simulink model "project"  (R2022b)
settings: Solver=ode15s  StartTime=0.0  StopTime=2  RelTol=1e-3
libraries: spsSeriesRLCBranchLib x6, spsVoltageMeasurementLib x4, spsCurrentMeasurementLib x3, spsFullBridgeMMCExternalDCLinksLib x1, spsOnDelayLib x1, spsPVArrayLib x1, spsPWMGeneratorMultilevelLib x1, spsDiodeLib x1, spsMosfetLib x1, spspowerguiLib x1
settings Model: Creator=nisha  LastModifiedBy=nisha

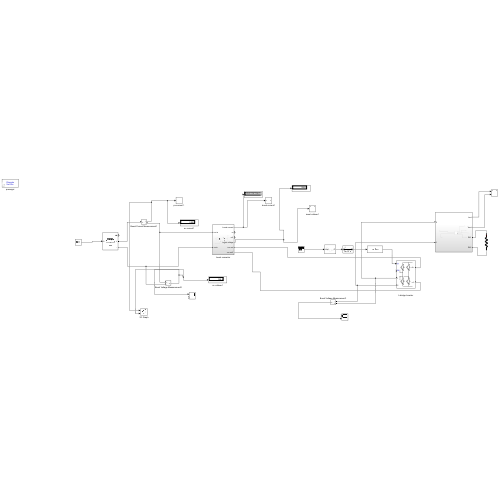
[thumbnail: Simulink's stored preview of the top-level diagram]
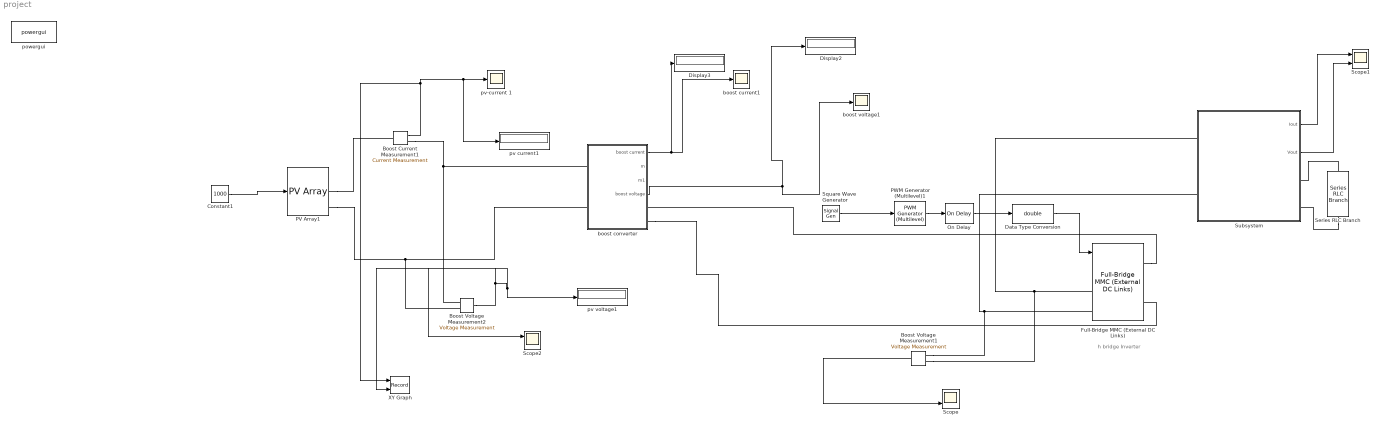
== system project ==
  note: h bridge Inverter
  Boost Current Measurement1 : spsCurrentMeasurementLib/Current Measurement  PhasorSimulation=off  OutputType=Complex  PSBequivalent=0
  Boost Voltage Measurement1 : spsVoltageMeasurementLib/Voltage Measurement  PhasorSimulation=off  OutputType=Complex  PSBequivalent=0
  Boost Voltage Measurement2 : spsVoltageMeasurementLib/Voltage Measurement  PhasorSimulation=off  OutputType=Complex  PSBequivalent=0
  Constant1 : Constant  Value=1000
  Data Type Conversion : DataTypeConversion  OutDataTypeStr=double  SaturateOnIntegerOverflow=off  RndMeth=Floor
  Display2 : Display
  Display3 : Display
      settings: Format=long_e
  Full-Bridge MMC (External DC Links) : spsFullBridgeMMCExternalDCLinksLib/Full-Bridge MMC (External DC Links)  ModelType=Switching devices  n=1  Ron=1e-3  Rs=1e6  Cs=inf  Ron_Diode=1e-3  Rs_Diode=1e6  Cs_Diode=inf  Vf_Diode=1e-3  Rs_CurrentSource=inf  Ts=10e-6
      settings: LibrarySourceBlock=|
      | sps_lib/Power Electronics/Full-Bridge MMC
      | (External DC Links)
  On Delay : spsOnDelayLib/On Delay  DelayType=On delay  delay=5e-7  ic=0  Ts=0
  PV Array1 : spsPVArrayLib/PV Array  Npar=1  Nser=5  PlotType=array @ 1000 W/m2 & specified temperatures  S_vec="[ 1000  500  100 ]"  Temp_C_vec="[ 45 25  ]"  ModuleName=User-defined  PlotWhenSelected=off  Pm=213.15  Ncell=60  Voc=36.3  Isc=7.84  Vm=29  Im=7.35  beta_Voc_pc=-0.36099  alpha_Isc_pc=0.102  beta_Voc=-0.13104  alpha_Isc=0.0079968  IL=7.8654  I0=2.9273e-10  nI=0.98119  Rsh=313.0553  Rs=0.39381  RobustModel=on  RobustCellTemperature=25  BAL=on  Tc=1e-6  Tfilter=5e-5
  PWM Generator (Multilevel)1 : spsPWMGeneratorMultilevelLib/PWM Generator (Multilevel)  BridgeType=Full-bridge  NumberOfBridges=1  Fc=540  Ts=0  ShowCarriersOutport=off
      settings: LibrarySourceBlock=|
      | sps_lib/Power Electronics/Power Electronics Control/PWM Generator
      | (Multilevel)
  Scope : Scope  NumInputPorts=2
  Scope1 : Scope  NumInputPorts=2
  Scope2 : Scope  NumInputPorts=2
  Series RLC Branch : spsSeriesRLCBranchLib/Series RLC Branch  LConnTagsString=__new0  RConnTagsString=__new0  BranchType=R  Resistance=110  Inductance=1e-3  SetiL0=off  InitialCurrent=0  Capacitance=1e-6  Setx0=off  InitialVoltage=0  Measurements=None
  Square Wave Generator : SignalGenerator  Frequency=2*pi*50  Units=rad/sec
  Subsystem : Subsystem
  XY Graph : Record  FileSettingsInternal="{\"entries\":[{\"content\":{\"excelSettings\":{\"content\":{},\"type\":\"Streamout.ExcelSettings\"}},\"type\":\"Streamout.FileSettingStorage\",\"uuid\":\"22b0a6b4-2c82-41ee-9664-83160f40e043\"}],\"packageUris\":[\"http://schema.mathworks.com/mf0/streamout_blocks/R2020a\"],\"version\":\"1.0\"}"  Layout=[1 1]  SignalsInternal="{\"entries\":[{\"content\":{\"signals\":[{\"content\":{\"blockPath\":[\"project/XY Graph\"],\"channel\":[],\"dimensions\":[1],\"domain\":\"project/XY Graph\",\"lineColor\":\"#a2142f\",\"plots\":[1],\"port\":1,\"sid\":[\"\"],\"signalID\":4156,\"signalName\":\"Boost Current Measurement1\"},\"type\":\"RecordBlkView.Signal\",\"uuid\":\"243745d2-b0e1-4b31-8906-84a58384e0b6\"},{\"content\":{\"blockPath\":[\"project/XY Graph\"],\"channel\":[],\"dimensions\":[1],\"domain\":\"project/XY Graph\",\"lineColor\":\"#139fff\",\"plots\":[1],\"port\":2,\"sid\":[\"\"],\"signalID\":4160,\"signalName\":\"Boost Voltage Measurement2\"},\"type\":\"RecordBlkView.Signal\",\"uuid\":\"0702fd03-a051-4114-9bf7-358e7a77b986\"}]},\"type\":\"RecordBlkView.InputSignals\",\"uuid\":\"78026cc8-cd91-4cf1-a118-0febc4990bc4\"}],\"packageUris\":[\"http://schema.mathworks.com/mf0/streamout_blocks/R2020a\"],\"version\":\"1.0\"}"  VisualizationBindings="{\"xyplotplugin\":{\"info\":[{\"series\":[{\"bindingParametersList\":[{\"parameter\":\"X-Axis\",\"signalID\":4156,\"signalName\":\"Boost Current Measurement1\"},{\"parameter\":\"Y-Axis\",\"signalID\":4160,\"signalName\":\"Boost Voltage Measurement2\"}],\"seriesID\":27621}],\"subplotID\":1}]}}"  CompatibilityTag=XY
  boost converter : Subsystem
  boost current1 : Scope
  boost voltage1 : Scope
  powergui : spspowerguiLib/powergui  Priority=1  SimulationMode=Discrete  SampleTime=5e-5  frequency=60  Iterations=50  frequencyindice=0  Pbase=100e6  ErrMax=1e-4  UnitsV=kV  UnitsW=MW  buscounter=0  FunctionMessages=off  echomessages=off  EnableUseOfTLC=off  CurrentSourceSwitches=off  DisableSnubberDevices=off  DisableRonSwitches=off  DisableVfSwitches=off  DisplayEquations=off  AutomaticDiscreteSolvers=off  SolverType=Tustin/Backward Euler (TBE)  Interpol=off  ExternalGateDelay=off  methode=off  Ts=100  x0status=blocks  SPID=on  SwTol=0  HookPort=off  NonlinearTolerance=1e-4  nMaxIteration=100  ContinueOnMaxIteration=off  RestoreLinks=warning  ResistiveCurrentMeasurement=off  Frange=[0:2:500]  Ylog=off  Xlog=on  ShowGrid=off  save=off  variable=ZData  structure=0  ZoomFFT=off  StartTime=0.0  cycles=1  DisplayStyle=1  fundamental=60  FreqAxis=off  MaxFrequency=1000  frequencyindicesteady=1  RmsSteady=1  display=off
  pv current1 : Display
  pv voltage1 : Display
  pv-current 1 : Scope
  wires:
  Subsystem/2(Vout) -> Scope1/2
  Subsystem/1(Iout) -> Scope1/1
  Boost Voltage Measurement1/1 -> Scope/2
  Square Wave Generator/1 -> PWM Generator (Multilevel)1/1
  PWM Generator (Multilevel)1/1 -> On Delay/1
  On Delay/1 -> Data Type Conversion/1
  Data Type Conversion/1 -> Full-Bridge MMC (External DC Links)/1
  boost converter/1(boost current) -> Display3/1, boost current1/1
  boost converter/4(boost voltage) -> boost voltage1/1, Display2/1
  Boost Voltage Measurement2/1 -> XY Graph/2, Scope2/1, pv voltage1/1
  Boost Current Measurement1/1 -> XY Graph/1, pv current1/1, pv-current 1/1
  Constant1/1 -> PV Array1/1
  connections:
  Series RLC Branch/LConn1 -- Subsystem/RConn1
  Series RLC Branch/RConn1 -- Subsystem/RConn2
  Boost Voltage Measurement1/LConn1 -- Full-Bridge MMC (External DC Links)/LConn1 -- Subsystem/LConn1
  Boost Voltage Measurement1/LConn2 -- Full-Bridge MMC (External DC Links)/LConn2 -- Subsystem/LConn2
  Full-Bridge MMC (External DC Links)/RConn1 -- boost converter/RConn1
  Boost Voltage Measurement2/LConn1 -- boost converter/LConn1 -- Boost Current Measurement1/RConn1
  Boost Voltage Measurement2/LConn2 -- boost converter/LConn2 -- PV Array1/RConn2
  PV Array1/RConn1 -- Boost Current Measurement1/LConn1
  boost converter/RConn2 -- Full-Bridge MMC (External DC Links)/RConn2

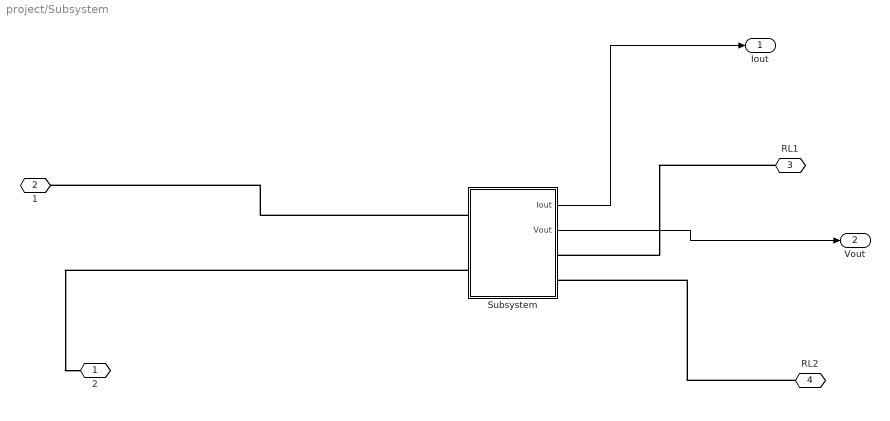
== system project/Subsystem ==
  Subsystem : Subsystem
  2 : PMIOPort  Side=Left
  1 : PMIOPort  Port=2  Side=Left
  RL1 : PMIOPort  Port=3  Side=Right
  RL2 : PMIOPort  Port=4  Side=Right
  Iout : Outport
  Vout : Outport  Port=2
  wires:
  Subsystem/1(Iout) -> Iout/1
  Subsystem/2(Vout) -> Vout/1
  connections:
  Subsystem/LConn1 -- 1/RConn1
  Subsystem/LConn2 -- 2/RConn1
  RL1/RConn1 -- Subsystem/RConn1
  RL2/RConn1 -- Subsystem/RConn2

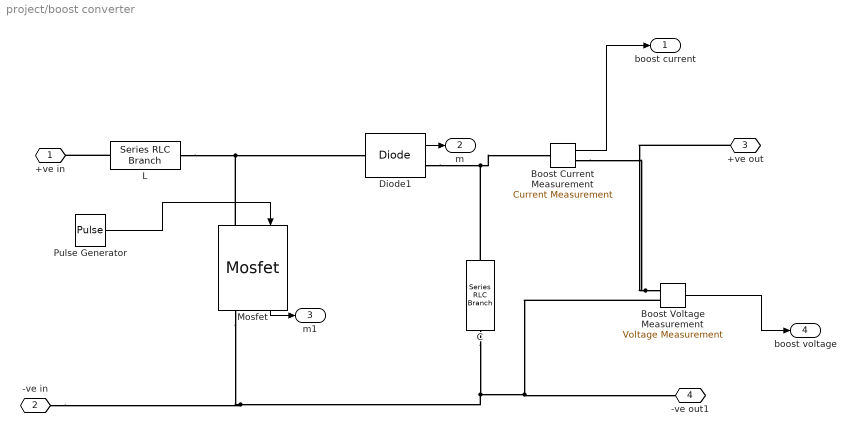
== system project/boost converter ==
  Boost Current Measurement : spsCurrentMeasurementLib/Current Measurement  PhasorSimulation=off  OutputType=Complex  PSBequivalent=0
  Boost Voltage Measurement : spsVoltageMeasurementLib/Voltage Measurement  PhasorSimulation=off  OutputType=Complex  PSBequivalent=0
  C : spsSeriesRLCBranchLib/Series RLC Branch  LConnTagsString=__new0  RConnTagsString=__new0  BranchType=C  Resistance=1e-3  Inductance=250e-6  SetiL0=off  InitialCurrent=0  Capacitance=1000e-6  Setx0=off  InitialVoltage=0  Measurements=None
  Diode1 : spsDiodeLib/Diode  Ron=0.001  Lon=0  Vf=0.8  IC=0  UseSnubber=0  Rs=500  Cs=250e-9  Measurements=on
  L : spsSeriesRLCBranchLib/Series RLC Branch  LConnTagsString=__new0  RConnTagsString=__new0  BranchType=L  Resistance=1e-3  Inductance=400e-3  SetiL0=off  InitialCurrent=0  Capacitance=1e-6  Setx0=off  InitialVoltage=0  Measurements=None
  Mosfet : spsMosfetLib/Mosfet  Ron=0.1  Lon=0  Rd=0.01  Vfd=0  IC=0  Rs=1e5  Cs=inf  Measurements=on
  Pulse Generator : DiscretePulseGenerator  PulseType=Time based  Period=1/10000  PulseWidth=20
  +ve in : PMIOPort  Side=Left
  -ve in : PMIOPort  Port=2  Side=Left
  +ve out : PMIOPort  Port=3  Side=Right
  -ve out1 : PMIOPort  Port=4  Side=Right
  boost current : Outport
  m : Outport  Port=2
  m1 : Outport  Port=3
  boost voltage : Outport  Port=4
  wires:
  Mosfet/1 -> m1/1
  Boost Current Measurement/1 -> boost current/1
  Pulse Generator/1 -> Mosfet/1
  Boost Voltage Measurement/1 -> boost voltage/1
  Diode1/1 -> m/1
  connections:
  Mosfet/LConn1 -- L/RConn1 -- Diode1/LConn1
  Diode1/RConn1 -- C/LConn1 -- Boost Current Measurement/LConn1
  -ve in/RConn1 -- Mosfet/RConn1 -- C/RConn1 -- Boost Voltage Measurement/LConn2 -- -ve out1/RConn1
  Boost Voltage Measurement/LConn1 -- Boost Current Measurement/RConn1 -- +ve out/RConn1
  L/LConn1 -- +ve in/RConn1

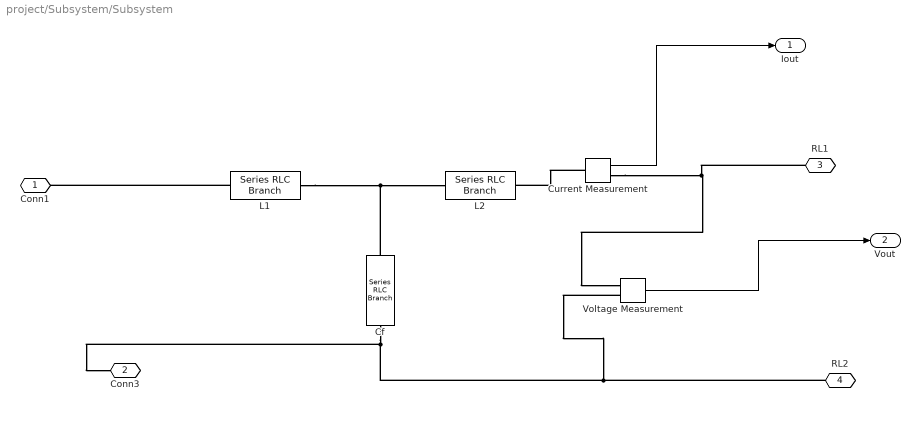
== system project/Subsystem/Subsystem ==
  Cf : spsSeriesRLCBranchLib/Series RLC Branch  LConnTagsString=__new0  RConnTagsString=__new0  BranchType=C  Resistance=1e-3  Inductance=400e-3  SetiL0=off  InitialCurrent=0  Capacitance=20e-6  Setx0=off  InitialVoltage=0  Measurements=None
  Current Measurement : spsCurrentMeasurementLib/Current Measurement  PhasorSimulation=off  OutputType=Complex  PSBequivalent=0
  L1 : spsSeriesRLCBranchLib/Series RLC Branch  LConnTagsString=__new0  RConnTagsString=__new0  BranchType=L  Resistance=1e-3  Inductance=50e-3  SetiL0=off  InitialCurrent=0  Capacitance=1e-6  Setx0=off  InitialVoltage=0  Measurements=None
  L2 : spsSeriesRLCBranchLib/Series RLC Branch  LConnTagsString=__new0  RConnTagsString=__new0  BranchType=L  Resistance=1e-3  Inductance=20e-3  SetiL0=off  InitialCurrent=0  Capacitance=1e-6  Setx0=off  InitialVoltage=0  Measurements=None
  Voltage Measurement : spsVoltageMeasurementLib/Voltage Measurement  PhasorSimulation=off  OutputType=Complex  PSBequivalent=0
  Conn1 : PMIOPort  Side=Left
  Conn3 : PMIOPort  Port=2  Side=Left
  RL1 : PMIOPort  Port=3  Side=Right
  RL2 : PMIOPort  Port=4  Side=Right
  Iout : Outport
  Vout : Outport  Port=2
  wires:
  Voltage Measurement/1 -> Vout/1
  Current Measurement/1 -> Iout/1
  connections:
  Current Measurement/LConn1 -- L2/RConn1
  Current Measurement/RConn1 -- RL1/RConn1 -- Voltage Measurement/LConn1
  Cf/RConn1 -- Conn3/RConn1 -- RL2/RConn1 -- Voltage Measurement/LConn2
  L1/RConn1 -- Cf/LConn1 -- L2/LConn1
  L1/LConn1 -- Conn1/RConn1
